simulink model "simulation"  (R2014a)
settings: Solver=ode45  StartTime=0.0  StopTime=10.0  RelTol=1e-3
settings Model: Creator=flp  LastModifiedBy=flp
settings DataIOCC: Refine=10

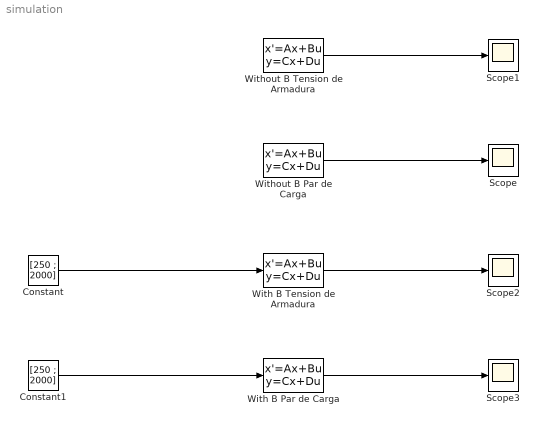
== system simulation ==
  Constant : Constant  Value=[250 ; 2000]
  Constant1 : Constant  Value=[250 ; 2000]
  Scope{,1..3} (4 alike) : Scope
      Scope1 settings: YMin=770  YMax=930
      Scope2 settings: SaveName=ScopeData2
      Scope3 settings: SaveName=ScopeData3
  "With B Par de Carga " : StateSpace  A=[-33.3 -7956 ; 0.1814 0]  B=[2.19298 0; 0 -0.05]  C=[0 1]  D=[0 0]  X0=[823 ; 105]
  "With B Tension de Armadura " : StateSpace  A=[-33.3 -7956 ; 0.1814 0]  B=[2.19298 0; 0 -0.05]  C=[1 0]  D=[0 0]  X0=[823 ; 105]
  "Without B Par de Carga " : StateSpace  A=[-33.3 -7956 ; 0.1814 0]  B="[0  0; 0 0]"  C=[0 1]  D=[0 0]  X0=[823 ; 105]
  Without B Tension de Armadura : StateSpace  A=[-33.3 -7956 ; 0.1814 0]  B="[0  0; 0 0]"  C=[1 1]  D=[0 0]  X0=[823 ; 105]
  wires:
  "Without B Par de Carga "/1 -> Scope/1
  "With B Tension de Armadura "/1 -> Scope2/1
  "With B Par de Carga "/1 -> Scope3/1
  Constant/1 -> "With B Tension de Armadura "/1
  Constant1/1 -> "With B Par de Carga "/1
  Without B Tension de Armadura/1 -> Scope1/1
